simulink model "xpc_osc3"  (Simulink 5.0)
settings: Solver=ode4  StartTime=0.0  StopTime=20  FixedStep=0.000250  RelTol=1e-3
libraries: xpclib x1
settings Model: Creator=mvetsch  LastModifiedBy=monchamp  RTWSystemTargetFile=xpctarget.tlc  RTWOptions="-aEnforceIntegerDowncast=0 -aExtMode=1 -aFoldNonRolledExpr=0 -aForceParamTrailComments=0 -aGenerateComments=1 -aGenerateReport=1 -aIncHierarchyInIds=0 -aInlineInvariantSignals=0 -aInlineParameters=0 -aLocalBlockOutputs=0 -aRL32IRQSourceModifier=\"Timer\" -aRL32LogBufSizeModifier=100000 -aRL32LogTETModifier=1 -aRL32ModeModifier=\"Real-Time\" -aRL32ObjectName=\"tg\" -aRTWVerbose=1 -aRollThreshold=5 -aShowEliminatedStatements=1 -axpcDblBuff=0 -axpcObjCom=0"  RTWTemplateMakefile=xpc_default_tmf  ExtModeMexFile=ext_xpc  ExtModeTrigMode=oneshot  ExtModeArmWhenConnect=off  SaveState=on  LimitDataPoints=off  BlockReductionOpt=off  BooleanDataType=off  OptimizeBlockIOStorage=off

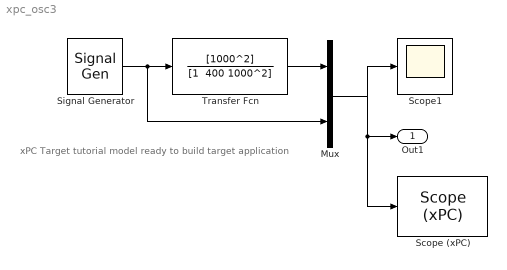
== system xpc_osc3 ==
  note: xPC Target tutorial model
      | ready to build target application
  Mux : Mux  Inputs=2
  "Scope (xPC) " : xpclib/Misc./Scope (xPC)   scopeno=1  scopetype=Target  viewmode=Graphical redraw  grid=on  ylimits=[0,0]  autostart=on  nosamples=500  noprepostsamples=0  interleave=1  triggermode=Signal Triggering  triggersignal=1  triggerlevel=0.0  triggerslope=rising  triggerscope=1
  Scope1 : Scope
      settings: TickLabels=on  TimeRange=0.2  YMin=-10  YMax=10  Decimation=2  SampleInput=on
  Signal Generator : SignalGenerator  WaveForm=square  Amplitude=4  Frequency=20
  Transfer Fcn : TransferFcn  Numerator=[1000^2]  Denominator="[1  400 1000^2]"
  Out1 : Outport
  wires:
  Signal Generator/1 -> Transfer Fcn/1, Mux/2
  Mux/1 -> Scope1/1, "Scope (xPC) "/1, Out1/1
  Transfer Fcn/1 -> Mux/1
